simulink library "uavsimBlockset_ManualLaw"  (Simulink 8.0)
settings: Solver=ode45  StartTime=0.0  StopTime=10.0  RelTol=1e-3
settings Model: Creator=mstolle  LastModifiedBy=j.bolting

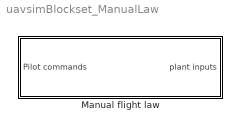
== system uavsimBlockset_ManualLaw ==
  Manual flight law : Subsystem  mask{mask_scale_da=0, mask_scale_de=0, mask_scale_dr=0, mask_scale_den=0, mask_scale_df=0, mask_utrim=0}
      mask prompts: mask_scale_da "Aileron command scale factor [rad]"; mask_scale_de "Elevator command scale factor [rad]"; mask_scale_dr "Rudder command scale factor [rad]"; mask_scale_den "Engine command scale factor [1]"; mask_scale_df "Flap command scale factor [rad]"; mask_utrim "Trim inputs [da de dr den df]"

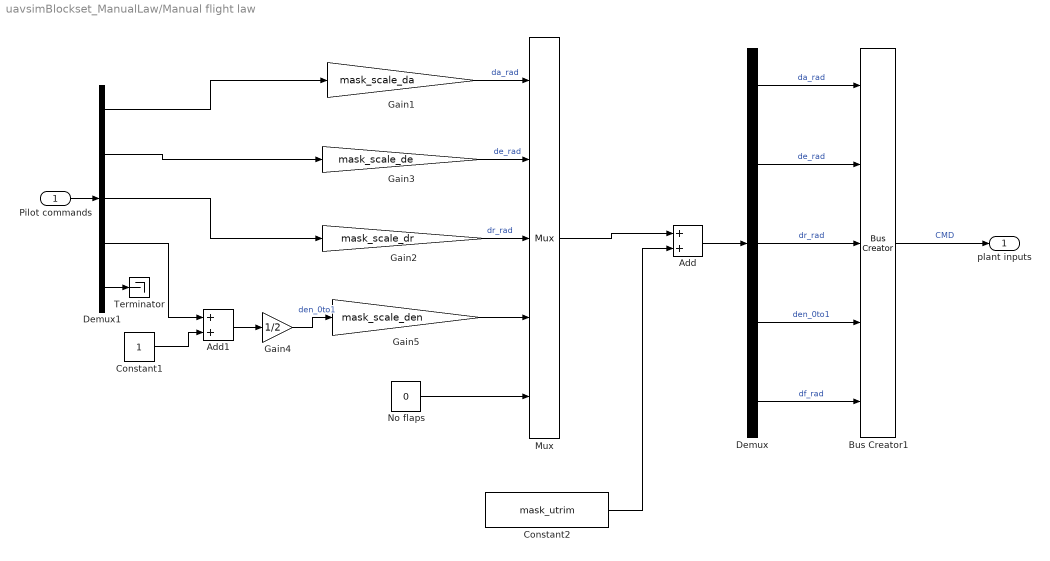
== system uavsimBlockset_ManualLaw/Manual flight law ==
  Pilot commands : Inport
  Add : Sum
  Add1 : Sum
  Bus Creator1 : BusCreator  Inputs=5  OutDataTypeStr=Bus: CMD  NonVirtualBus=on
  Constant1 : Constant
  Constant2 : Constant  Value=mask_utrim
  Demux : Demux  Outputs=5
  Demux1 : Demux  Outputs=[1 1 1 1 6]
  Gain1 : Gain  Gain=mask_scale_da
  Gain2 : Gain  Gain=mask_scale_dr
  Gain3 : Gain  Gain=mask_scale_de
  Gain4 : Gain  Gain=1/2
  Gain5 : Gain  Gain=mask_scale_den
  Mux : Mux  Inputs=5
  No flaps : Constant  Value=0
  Terminator : Terminator
  plant inputs : Outport  OutDataTypeStr=Bus: CMD
  wires:
  Demux1/5 -> Terminator/1
  Pilot commands/1 -> Demux1/1
  Add1/1 -> Gain4/1
  Demux1/4 -> Add1/1
  Constant1/1 -> Add1/2
  Demux1/2 -> Gain3/1
  Demux/2 -> Bus Creator1/2  "de_rad"
  Demux/1 -> Bus Creator1/1  "da_rad"
  Demux/4 -> Bus Creator1/4  "den_0to1"
  Demux/3 -> Bus Creator1/3  "dr_rad"
  Gain2/1 -> Mux/3  "dr_rad"
  Gain3/1 -> Mux/2  "de_rad"
  Gain1/1 -> Mux/1  "da_rad"
  Demux1/1 -> Gain1/1
  Demux1/3 -> Gain2/1
  Bus Creator1/1 -> plant inputs/1  "CMD"
  Mux/1 -> Add/1
  Demux/5 -> Bus Creator1/5  "df_rad"
  Gain4/1 -> Gain5/1  "den_0to1"
  Gain5/1 -> Mux/4
  Constant2/1 -> Add/2
  Add/1 -> Demux/1
  No flaps/1 -> Mux/5
